simulink model "walnut_1.0"  (R2022a)
settings: Solver=FixedStepAuto  StartTime=0.0  StopTime=inf  RelTol=1e-3
model workspace (MAT data in the model file):
  SL_ROS_VariableLengthArrays_MaxSizes.CommonInfo.ArrayTruncateAction = 'EmitWarning'
  SL_ROS_VariableLengthArrays_MaxSizes.MsgTypeMap = containers.Map
  SL_ROS_VariableLengthArrays_MaxSizes.MsgTypeMap.serialization.keys = {'std_msgs/Float32MultiArray'}
  SL_ROS_VariableLengthArrays_MaxSizes.MsgTypeMap.serialization.values{1}.PropertyName = 'Data'
  SL_ROS_VariableLengthArrays_MaxSizes.MsgTypeMap.serialization.values{1}.DataType = 'single'
  SL_ROS_VariableLengthArrays_MaxSizes.MsgTypeMap.serialization.values{1}.MaxLength = 4
  SL_ROS_VariableLengthArrays_MaxSizes.MsgTypeMap.serialization.uniformity = 0
  SL_ROS_VariableLengthArrays_MaxSizes.MsgTypeMap.serialization.keyType = 'char'
  SL_ROS_VariableLengthArrays_MaxSizes.MsgTypeMap.serialization.valueType = 'any'
  dq0 = [0; 0; 0; 0]
  q0 = [0; 0; 0; 0]
  robotToTest : robotics.RigidBodyTree (value not decoded)
undefined symbols (not defined in the file or in its folder): sawyer, X, Y, Z
libraries: sm_lib x105, nesl_utility x46, robotlib x13, robotmaniplib x6, simulink x5
(part 1 of 3)
settings Model: Creator=conno  LastModifiedBy=conno
settings OptimizationCC: EnhancedBackFolding=on  PassReuseOutputArgsAs=Individual arguments  ZeroExternalMemoryAtStartup=off  ZeroInternalMemoryAtStartup=off  MaxStackSize=64  OptimizeBlockOrder=speed  DifferentSizesBufferReuse=on  OptimizationCustomize=off  EfficientTunableParamExpr=on
settings DebuggingCC: ParameterTunabilityLossMsg=error
settings HardwareCC: ProdBitPerPointer=32  ProdBitPerSizeT=32  ProdBitPerPtrDiffT=32  ProdLargestAtomicFloat=None  ProdIntDivRoundTo=Undefined  ProdEndianess=Unspecified  ProdWordSize=32  ProdHWDeviceType=Generic->Unspecified (assume 32-bit Generic)  UseEmbeddedCoderFeatures=off
settings RTWCC: SystemTargetFile=ert.tlc  HardwareBoard=Robot Operating System (ROS)  TLCOptions="-aInlineSetEventsForThisBaseRateFcn=TLC_FALSE -aSuppressMultiTaskScheduler=TLC_FALSE  -aRateBasedStepFcn=0"  TemplateMakefile=ert_default_tmf  Toolchain=Catkin  TargetLang=C++
settings CodeAppCC: ForceParamTrailComments=on  IgnoreCustomStorageClasses=off  OperatorAnnotations=on  SimulinkDataObjDesc=on  SFDataObjDesc=on  InsertBlockDesc=on
settings ERTTargetCC: SupportNonInlinedSFcns=on

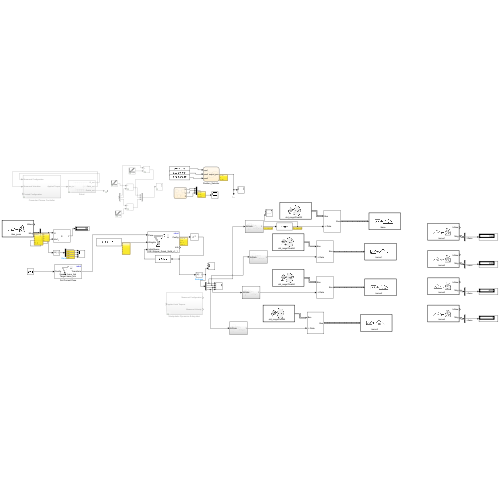
[thumbnail: Simulink's stored preview of the top-level diagram]
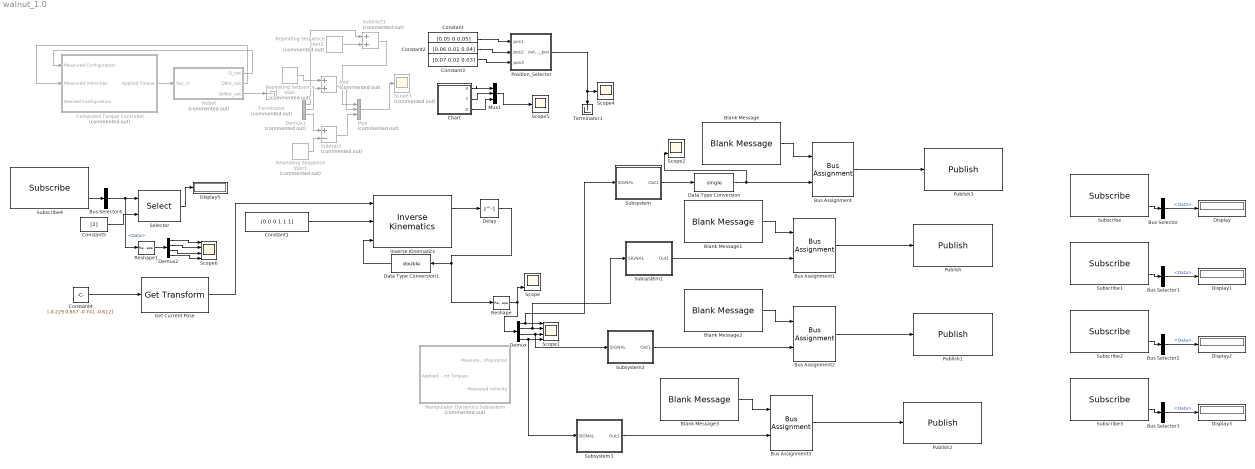
== system walnut_1.0 ==
  Add : Sum  Commented=on
  Blank Message : robotlib/Blank Message  messageClass=Message  entityType=std_msgs/Float32  messageType=std_msgs/Float32  SampleTime=inf  legacyBusStruct=off
  Blank Message1 : robotlib/Blank Message  messageClass=Message  entityType=std_msgs/Float64  messageType=std_msgs/Float64  SampleTime=inf  legacyBusStruct=off
  Blank Message2 : robotlib/Blank Message  messageClass=Message  entityType=std_msgs/Float64  messageType=std_msgs/Float64  SampleTime=inf  legacyBusStruct=off
  Blank Message3 : robotlib/Blank Message  messageClass=Message  entityType=std_msgs/Float64  messageType=std_msgs/Float64  SampleTime=inf  legacyBusStruct=off
  Bus Assignment{,1..3} (4 alike) : BusAssignment  AssignedSignals=Data
  Bus Selector{,1..4} (5 alike) : BusSelector  OutputSignals=Data
  Chart : Stateflow chart  TreatAsAtomicUnit=on
  Computed Torque Controller : Subsystem  Commented=on
  Constant : Constant  Value=[0.05 0 0.05]
  Constant1 : Constant  Value=[0 0 0 1 1 1]
  Constant2 : Constant  Value=[0.06 0.01 0.04]
  Constant3 : Constant  Value=[0.07 0.02 0.03]
  Constant4 : Constant  Value=[-0.229 0.857 -0.741 -0.612]
  Constant5 : Constant  Value=[2]
  Data Type Conversion : DataTypeConversion  OutDataTypeStr=single  SaturateOnIntegerOverflow=off  RndMeth=Floor
  Data Type Conversion1 : DataTypeConversion  OutDataTypeStr=double  SaturateOnIntegerOverflow=off  RndMeth=Floor
  Delay : Delay  DelayLength=1  InitialCondition=q0
  Demux : Demux
  Demux1 : Demux  Commented=on  Outputs=3
  Demux2 : Demux
  Display{,1..3,5} (5 alike) : Display
  Get Current Pose : robotmaniplib/Get Transform  RigidBodyTree=robot  SourceBody=base_link  TargetBody=base_link  SimulateUsing=Interpreted execution
  Inverse Kinematics : robotmaniplib/Inverse Kinematics  RigidBodyTree=robot  EndEffector=Gripper_Dumb_Solid_v1_1  ShowInfo=on  SolverName=BFGS Gradient Projection  EnforceJointLimits=on  MaxIterations=1500  MaxTime=10  GradientTolerance=1e-7  SolutionTolerance=1e-6  StepTolerance=1e-14  ErrorChangeTolerance=1e-12  UseErrorDamping=on  DampingBias=0.0025  SimulateUsing=Interpreted execution
  Manipulator Dynamics Subsystem : Subsystem  Commented=on
  Mux : Mux  Commented=on  Inputs=3
  Mux1 : Mux  Inputs=3
  Position_Selector : Stateflow chart  TreatAsAtomicUnit=on
  Publish : robotlib/Publish  topicSource=Specify your own  topic=/servo1  messageType=std_msgs/Float64  legacyBusStruct=off  messageQueueLength=1
  Publish1 : robotlib/Publish  topicSource=Specify your own  topic=/servo2  messageType=std_msgs/Float64  legacyBusStruct=off  messageQueueLength=1
  Publish2 : robotlib/Publish  topicSource=Specify your own  topic=/servo3  messageType=std_msgs/Float64  legacyBusStruct=off  messageQueueLength=1
  Publish3 : robotlib/Publish  topicSource=Specify your own  topic=/base  messageType=std_msgs/Float32  legacyBusStruct=off  messageQueueLength=1
  Repeating Sequence Stair : simulink/Sources/Repeating Sequence Stair  Commented=on  OutValues=[0 0.01 0.02 0.03].'  tsamp=2  OutMin=[]  OutMax=[]  OutDataTypeStr=double  OutputDataTypeScalingMode=double  OutDataType=fixdt(0,8)  ConRadixGroup=Best Precision: Vector-wise  OutScaling=2^-12
  Repeating Sequence Stair1 : simulink/Sources/Repeating Sequence Stair  Commented=on  OutValues=[0 0.01 0.02 0.03].'  tsamp=2  OutMin=[]  OutMax=[]  OutDataTypeStr=double  OutputDataTypeScalingMode=double  OutDataType=fixdt(0,8)  ConRadixGroup=Best Precision: Vector-wise  OutScaling=2^-12
  Repeating Sequence Stair2 : simulink/Sources/Repeating Sequence Stair  Commented=on  OutValues=[0 0.01 0.02 0.03].'  tsamp=2  OutMin=[]  OutMax=[]  OutDataTypeStr=double  OutputDataTypeScalingMode=double  OutDataType=fixdt(0,8)  ConRadixGroup=Best Precision: Vector-wise  OutScaling=2^-12
  Reshape : Reshape
  Reshape1 : Reshape
  Robot : Subsystem  Commented=on
  Scope : Scope  NumInputPorts=3
  Scope1 : Scope  NumInputPorts=4
  Scope2 : Scope  NumInputPorts=3
  Scope3 : Scope  Commented=on
  Scope4 : Scope
  Scope5 : Scope
  Scope6 : Scope  NumInputPorts=4
  Selector : Selector  IndexOptions=Index vector (port)  Indices=[2]  OutputSizes=1
  Subscribe : robotlib/Subscribe  topicSource=Specify your own  topic=/servo1  messageType=std_msgs/Float64  SampleTime=-1  legacyBusStruct=off  messageQueueLength=1
  Subscribe1 : robotlib/Subscribe  topicSource=Specify your own  topic=/servo2  messageType=std_msgs/Float64  SampleTime=-1  legacyBusStruct=off  messageQueueLength=1
  Subscribe2 : robotlib/Subscribe  topicSource=Specify your own  topic=/servo3  messageType=std_msgs/Float64  SampleTime=-1  legacyBusStruct=off  messageQueueLength=1
  Subscribe3 : robotlib/Subscribe  topicSource=Specify your own  topic=/servo4  messageType=std_msgs/Float64  SampleTime=-1  legacyBusStruct=off  messageQueueLength=1
  Subscribe4 : robotlib/Subscribe  topicSource=Select from ROS network  topic=/des_pose  messageType=std_msgs/Float32MultiArray  SampleTime=-1  legacyBusStruct=off  messageQueueLength=1
  Subsystem : Subsystem
  Subsystem1 : Subsystem
  Subsystem2 : Subsystem
  Subsystem3 : Subsystem
  Subtract : Sum  Commented=on  Inputs=+-
  Subtract1 : Sum  Commented=on
  Terminator : Terminator  Commented=on
  Terminator1 : Terminator
  wires:
  Bus Selector3/1 -> Display3/1  "<Data>"
  Subscribe3/2 -> Bus Selector3/1
  Subscribe1/2 -> Bus Selector1/1
  Reshape/1 -> Scope/3, Demux/1
  Computed Torque Controller/1(Applied Torque) -> Robot/1(tau_in)
  Demux/1 -> Subsystem/1(SIGNAL), Scope1/1
  Bus Assignment2/1 -> Publish1/1
  Blank Message1/1 -> Bus Assignment1/1
  Blank Message2/1 -> Bus Assignment2/1
  Bus Assignment1/1 -> Publish/1
  Bus Assignment3/1 -> Publish2/1
  Subscribe2/2 -> Bus Selector2/1
  Bus Selector2/1 -> Display2/1  "<Data>"
  Get Current Pose/1 -> Inverse Kinematics/1
  Inverse Kinematics/1 -> Delay/1
  Bus Selector/1 -> Display/1  "<Data>"
  Subscribe/2 -> Bus Selector/1
  Blank Message3/1 -> Bus Assignment3/1
  Demux/4 -> Subsystem3/1(SIGNAL), Scope1/4
  Robot/1(Q_out) -> Computed Torque Controller/1(Measured Configuration)
  Bus Selector1/1 -> Display1/1  "<Data>"
  Constant1/1 -> Inverse Kinematics/2
  Demux/3 -> Subsystem2/1(SIGNAL), Scope1/3
  Bus Assignment/1 -> Publish3/1
  Demux/2 -> Subsystem1/1(SIGNAL), Scope1/2
  Robot/2(Qdot_out) -> Computed Torque Controller/2(Measured Velocities)
  Robot/3(Qddot_out) -> Terminator/1
  Blank Message/1 -> Bus Assignment/1
  Delay/1 -> Reshape/1, Data Type Conversion1/1
  Subsystem/1(Out1) -> Data Type Conversion/1
  Subsystem1/1(Out1) -> Bus Assignment1/2
  Subsystem2/1(Out1) -> Bus Assignment2/2
  Subsystem3/1(Out1) -> Bus Assignment3/2
  Repeating Sequence Stair/1 -> Add/1
  Add/1 -> Mux/2
  Mux/1 -> Scope3/1
  Demux1/1 -> Subtract1/1
  Demux1/2 -> Add/2
  Demux1/3 -> Subtract/1
  Repeating Sequence Stair1/1 -> Subtract/2
  Subtract/1 -> Mux/3
  Repeating Sequence Stair2/1 -> Subtract1/2
  Subtract1/1 -> Mux/1
  Constant/1 -> Position_Selector/1(pos1)
  Constant2/1 -> Position_Selector/2(pos2)
  Constant3/1 -> Position_Selector/3(pos3)
  Position_Selector/1(output_pos) -> Terminator1/1, Scope4/1
  Chart/1(X) -> Mux1/1
  Chart/2(Y) -> Mux1/2
  Chart/3(Z) -> Mux1/3
  Mux1/1 -> Scope5/1
  Data Type Conversion/1 -> Scope2/3, Bus Assignment/2
  Data Type Conversion1/1 -> Inverse Kinematics/3
  Constant4/1 -> Get Current Pose/1
  Subscribe4/2 -> Bus Selector4/1
  Bus Selector4/1 -> Reshape1/1, Selector/1  "<Data>"
  Constant5/1 -> Selector/2
  Selector/1 -> Display5/1
  Demux2/1 -> Scope6/1
  Demux2/2 -> Scope6/2
  Demux2/3 -> Scope6/3
  Demux2/4 -> Scope6/4
  Reshape1/1 -> Demux2/1

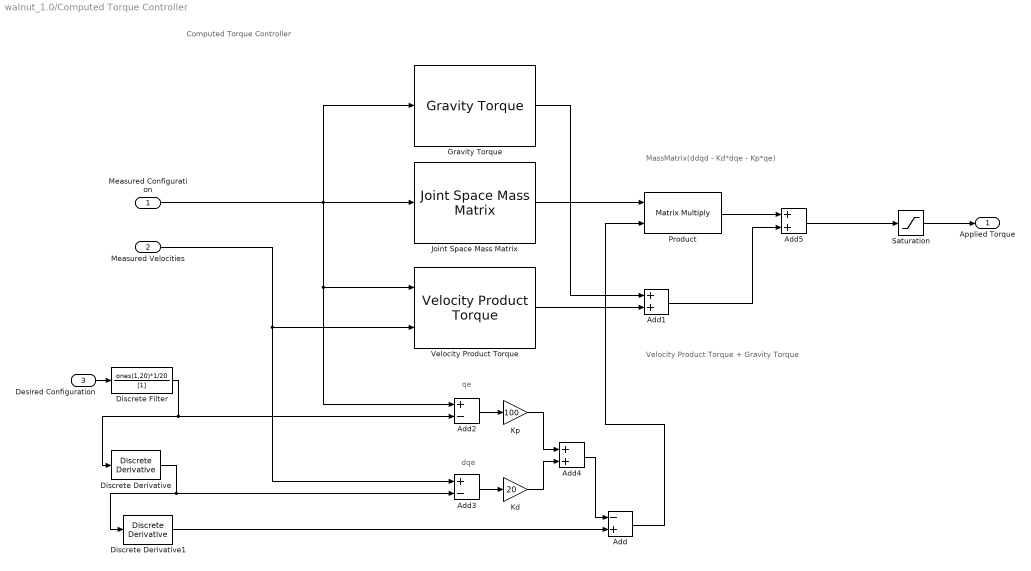
== system walnut_1.0/Computed Torque Controller ==
  note: Computed Torque Controller
  note: MassMatrix(ddqd - Kd*dqe - Kp*qe)
  note: Velocity Product Torque + Gravity Torque
  note: dqe
  note: qe
  Measured Configuration : Inport
  Measured Velocities : Inport  Port=2
  Desired Configuration : Inport  Port=3
  Add : Sum  Inputs=-+
  Add1 : Sum
  Add2 : Sum  Inputs=+-
  Add3 : Sum  Inputs=+-
  Add4 : Sum
  Add5 : Sum
  Discrete Derivative : simulink/Discrete/Discrete Derivative  gainval=1.0  ICPrevScaledInput=0.0  OutMin=[]  OutMax=[]  OutDataType=fixdt(1, 16)  OutScaling=2^-10  DoSatur=off
  Discrete Derivative1 : simulink/Discrete/Discrete Derivative  gainval=1.0  ICPrevScaledInput=0.0  OutMin=[]  OutMax=[]  OutDataType=fixdt(1, 16)  OutScaling=2^-10  DoSatur=off
  Discrete Filter : DiscreteFilter  Numerator=ones(1,20)*1/20  Denominator=[1]  InitialStates=repmat(q0',19,1)
  Gravity Torque : robotmaniplib/Gravity Torque  RigidBodyTree=robot  SimulateUsing=Interpreted execution
  Joint Space Mass Matrix : robotmaniplib/Joint Space Mass Matrix  RigidBodyTree=robot  SimulateUsing=Interpreted execution
  Kd : Gain  Gain=20
  Kp : Gain  Gain=100
  Product : Product  Multiplication=Matrix(*)
  Saturation : Saturate  UpperLimit=100  LowerLimit=-100
  Velocity Product Torque : robotmaniplib/Velocity Product Torque  RigidBodyTree=robot  SimulateUsing=Interpreted execution
      settings: SourceProductBaseCode=RO
  Applied Torque : Outport  VectorParamsAs1DForOutWhenUnconnected=off
  wires:
  Saturation/1 -> Applied Torque/1
  Velocity Product Torque/1 -> Add1/2
  Gravity Torque/1 -> Add1/1
  Add1/1 -> Add5/2
  Product/1 -> Add5/1
  Add5/1 -> Saturation/1
  Kd/1 -> Add4/2
  Kp/1 -> Add4/1
  Add3/1 -> Kd/1
  Add2/1 -> Kp/1
  Discrete Derivative/1 -> Discrete Derivative1/1, Add3/2
  Desired Configuration/1 -> Discrete Filter/1
  Add/1 -> Product/2
  Discrete Derivative1/1 -> Add/2
  Add4/1 -> Add/1
  Measured Velocities/1 -> Velocity Product Torque/2, Add3/1
  Measured Configuration/1 -> Add2/1, Velocity Product Torque/1, Gravity Torque/1, Joint Space Mass Matrix/1
  Joint Space Mass Matrix/1 -> Product/1
  Discrete Filter/1 -> Discrete Derivative/1, Add2/2

== system walnut_1.0/Manipulator Dynamics Subsystem ==
  Applied Joint Torques : Inport
  Integrator : Integrator
  Integrator1 : Integrator  InitialCondition=q0
  Manipulator Dynamics Model : robotmaniplib/Forward Dynamics  RigidBodyTree=robot  SimulateUsing=Interpreted execution
  Zero : Constant  Value=zeros(6, sawyer.NumBodies)  OutDataTypeStr=Inherit: Inherit via back propagation
  Measured Configuration : Outport  VectorParamsAs1DForOutWhenUnconnected=off
  Measured Velocity : Outport  Port=2  VectorParamsAs1DForOutWhenUnconnected=off
  wires:
  Integrator1/1 -> Manipulator Dynamics Model/1, Measured Configuration/1
  Manipulator Dynamics Model/1 -> Integrator/1
  Integrator/1 -> Integrator1/1, Manipulator Dynamics Model/2, Measured Velocity/1
  Applied Joint Torques/1 -> Manipulator Dynamics Model/3
  Zero/1 -> Manipulator Dynamics Model/4

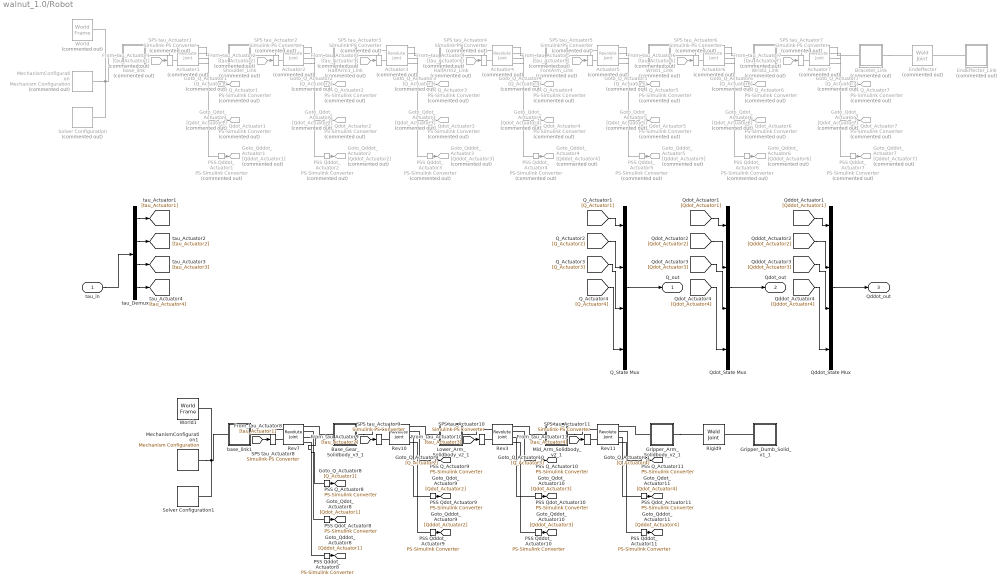
== system walnut_1.0/Robot ==
  tau_in : Inport
  Actuator1 : sm_lib/Joints/Revolute Joint  Commented=on  JointMode=Normal  SenseConstraintForce=off  SenseConstraintForceX=off  SenseConstraintForceY=off  SenseConstraintForceZ=off  SenseConstraintTorque=off  SenseConstraintTorqueX=off  SenseConstraintTorqueY=off  SenseConstraintTorqueZ=off  SenseTotalForce=off  SenseTotalForceX=off  SenseTotalForceY=off  SenseTotalForceZ=off  SenseTotalTorque=off  SenseTotalTorqueX=off  SenseTotalTorqueY=off  SenseTotalTorqueZ=off  CompositeWrenchDir=FollowerOnBase  CompositeWrenchFrame=BaseFrame  EquilibriumPosition=0  EquilibriumPositionUnits=deg  SpringStiffness=0  SpringStiffnessUnits=N*m/deg  DampingCoefficient=0  DampingCoefficientUnits=kg*m^2/(rad*s)  TorqueActuationMode=InputTorque  MotionActuationMode=ComputedMotion  SensePosition=on  SenseVelocity=on  SenseAcceleration=on  SenseTorqueForce=off  SenseLowerLimitTorqueForce=off  SenseUpperLimitTorqueForce=off  LowerLimitSpecify=off  LowerLimitBound=-90  LowerLimitBoundUnits=deg  LowerLimitStiffness=1e4  LowerLimitStiffnessUnits=N*m/deg  LowerLimitDamping=10  LowerLimitDampingUnits=N*m/(deg/s)  LowerLimitTransitionRegionWidth=0.1  LowerLimitTransitionRegionWidthUnits=deg  UpperLimitSpecify=off  UpperLimitBound=90  UpperLimitBoundUnits=deg  UpperLimitStiffness=1e4  UpperLimitStiffnessUnits=N*m/deg  UpperLimitDamping=10  UpperLimitDampingUnits=N*m/(deg/s)  UpperLimitTransitionRegionWidth=0.1  UpperLimitTransitionRegionWidthUnits=deg  PositionTargetSpecify=on  PositionTargetPriority=High  PositionTargetValue=q0(1)  PositionTargetValueUnits=rad  VelocityTargetSpecify=on  VelocityTargetPriority=High  VelocityTargetValue=dq0(1)  VelocityTargetValueUnits=rad/s
  Actuator2 : sm_lib/Joints/Revolute Joint  Commented=on  JointMode=Normal  SenseConstraintForce=off  SenseConstraintForceX=off  SenseConstraintForceY=off  SenseConstraintForceZ=off  SenseConstraintTorque=off  SenseConstraintTorqueX=off  SenseConstraintTorqueY=off  SenseConstraintTorqueZ=off  SenseTotalForce=off  SenseTotalForceX=off  SenseTotalForceY=off  SenseTotalForceZ=off  SenseTotalTorque=off  SenseTotalTorqueX=off  SenseTotalTorqueY=off  SenseTotalTorqueZ=off  CompositeWrenchDir=FollowerOnBase  CompositeWrenchFrame=BaseFrame  EquilibriumPosition=0  EquilibriumPositionUnits=deg  SpringStiffness=0  SpringStiffnessUnits=N*m/deg  DampingCoefficient=0  DampingCoefficientUnits=kg*m^2/(rad*s)  TorqueActuationMode=InputTorque  MotionActuationMode=ComputedMotion  SensePosition=on  SenseVelocity=on  SenseAcceleration=on  SenseTorqueForce=off  SenseLowerLimitTorqueForce=off  SenseUpperLimitTorqueForce=off  LowerLimitSpecify=on  LowerLimitBound=-2.2  LowerLimitBoundUnits=rad  LowerLimitStiffness=1e4  LowerLimitStiffnessUnits=N*m/deg  LowerLimitDamping=10  LowerLimitDampingUnits=N*m/(deg/s)  LowerLimitTransitionRegionWidth=0.1  LowerLimitTransitionRegionWidthUnits=deg  UpperLimitSpecify=on  UpperLimitBound=2.2  UpperLimitBoundUnits=rad  UpperLimitStiffness=1e4  UpperLimitStiffnessUnits=N*m/deg  UpperLimitDamping=10  UpperLimitDampingUnits=N*m/(deg/s)  UpperLimitTransitionRegionWidth=0.1  UpperLimitTransitionRegionWidthUnits=deg  PositionTargetSpecify=on  PositionTargetPriority=High  PositionTargetValue=q0(2)  PositionTargetValueUnits=rad  VelocityTargetSpecify=on  VelocityTargetPriority=High  VelocityTargetValue=dq0(2)  VelocityTargetValueUnits=rad/s
  Actuator3 : sm_lib/Joints/Revolute Joint  Commented=on  JointMode=Normal  SenseConstraintForce=off  SenseConstraintForceX=off  SenseConstraintForceY=off  SenseConstraintForceZ=off  SenseConstraintTorque=off  SenseConstraintTorqueX=off  SenseConstraintTorqueY=off  SenseConstraintTorqueZ=off  SenseTotalForce=off  SenseTotalForceX=off  SenseTotalForceY=off  SenseTotalForceZ=off  SenseTotalTorque=off  SenseTotalTorqueX=off  SenseTotalTorqueY=off  SenseTotalTorqueZ=off  CompositeWrenchDir=FollowerOnBase  CompositeWrenchFrame=BaseFrame  EquilibriumPosition=0  EquilibriumPositionUnits=deg  SpringStiffness=0  SpringStiffnessUnits=N*m/deg  DampingCoefficient=0  DampingCoefficientUnits=kg*m^2/(rad*s)  TorqueActuationMode=InputTorque  MotionActuationMode=ComputedMotion  SensePosition=on  SenseVelocity=on  SenseAcceleration=on  SenseTorqueForce=off  SenseLowerLimitTorqueForce=off  SenseUpperLimitTorqueForce=off  LowerLimitSpecify=off  LowerLimitBound=-90  LowerLimitBoundUnits=deg  LowerLimitStiffness=1e4  LowerLimitStiffnessUnits=N*m/deg  LowerLimitDamping=10  LowerLimitDampingUnits=N*m/(deg/s)  LowerLimitTransitionRegionWidth=0.1  LowerLimitTransitionRegionWidthUnits=deg  UpperLimitSpecify=off  UpperLimitBound=90  UpperLimitBoundUnits=deg  UpperLimitStiffness=1e4  UpperLimitStiffnessUnits=N*m/deg  UpperLimitDamping=10  UpperLimitDampingUnits=N*m/(deg/s)  UpperLimitTransitionRegionWidth=0.1  UpperLimitTransitionRegionWidthUnits=deg  PositionTargetSpecify=on  PositionTargetPriority=High  PositionTargetValue=q0(3)  PositionTargetValueUnits=rad  VelocityTargetSpecify=on  VelocityTargetPriority=High  VelocityTargetValue=dq0(3)  VelocityTargetValueUnits=rad/s
  Actuator4 : sm_lib/Joints/Revolute Joint  Commented=on  JointMode=Normal  SenseConstraintForce=off  SenseConstraintForceX=off  SenseConstraintForceY=off  SenseConstraintForceZ=off  SenseConstraintTorque=off  SenseConstraintTorqueX=off  SenseConstraintTorqueY=off  SenseConstraintTorqueZ=off  SenseTotalForce=off  SenseTotalForceX=off  SenseTotalForceY=off  SenseTotalForceZ=off  SenseTotalTorque=off  SenseTotalTorqueX=off  SenseTotalTorqueY=off  SenseTotalTorqueZ=off  CompositeWrenchDir=FollowerOnBase  CompositeWrenchFrame=BaseFrame  EquilibriumPosition=0  EquilibriumPositionUnits=deg  SpringStiffness=0  SpringStiffnessUnits=N*m/deg  DampingCoefficient=0  DampingCoefficientUnits=kg*m^2/(rad*s)  TorqueActuationMode=InputTorque  MotionActuationMode=ComputedMotion  SensePosition=on  SenseVelocity=on  SenseAcceleration=on  SenseTorqueForce=off  SenseLowerLimitTorqueForce=off  SenseUpperLimitTorqueForce=off  LowerLimitSpecify=on  LowerLimitBound=-2.5656  LowerLimitBoundUnits=rad  LowerLimitStiffness=1e4  LowerLimitStiffnessUnits=N*m/deg  LowerLimitDamping=10  LowerLimitDampingUnits=N*m/(deg/s)  LowerLimitTransitionRegionWidth=0.1  LowerLimitTransitionRegionWidthUnits=deg  UpperLimitSpecify=on  UpperLimitBound=2.5656  UpperLimitBoundUnits=rad  UpperLimitStiffness=1e4  UpperLimitStiffnessUnits=N*m/deg  UpperLimitDamping=10  UpperLimitDampingUnits=N*m/(deg/s)  UpperLimitTransitionRegionWidth=0.1  UpperLimitTransitionRegionWidthUnits=deg  PositionTargetSpecify=on  PositionTargetPriority=High  PositionTargetValue=q0(4)  PositionTargetValueUnits=rad  VelocityTargetSpecify=on  VelocityTargetPriority=High  VelocityTargetValue=dq0(4)  VelocityTargetValueUnits=rad/s
  Actuator5 : sm_lib/Joints/Revolute Joint  Commented=on  JointMode=Normal  SenseConstraintForce=off  SenseConstraintForceX=off  SenseConstraintForceY=off  SenseConstraintForceZ=off  SenseConstraintTorque=off  SenseConstraintTorqueX=off  SenseConstraintTorqueY=off  SenseConstraintTorqueZ=off  SenseTotalForce=off  SenseTotalForceX=off  SenseTotalForceY=off  SenseTotalForceZ=off  SenseTotalTorque=off  SenseTotalTorqueX=off  SenseTotalTorqueY=off  SenseTotalTorqueZ=off  CompositeWrenchDir=FollowerOnBase  CompositeWrenchFrame=BaseFrame  EquilibriumPosition=0  EquilibriumPositionUnits=deg  SpringStiffness=0  SpringStiffnessUnits=N*m/deg  DampingCoefficient=0  DampingCoefficientUnits=kg*m^2/(rad*s)  TorqueActuationMode=InputTorque  MotionActuationMode=ComputedMotion  SensePosition=on  SenseVelocity=on  SenseAcceleration=on  SenseTorqueForce=off  SenseLowerLimitTorqueForce=off  SenseUpperLimitTorqueForce=off  LowerLimitSpecify=off  LowerLimitBound=-90  LowerLimitBoundUnits=deg  LowerLimitStiffness=1e4  LowerLimitStiffnessUnits=N*m/deg  LowerLimitDamping=10  LowerLimitDampingUnits=N*m/(deg/s)  LowerLimitTransitionRegionWidth=0.1  LowerLimitTransitionRegionWidthUnits=deg  UpperLimitSpecify=off  UpperLimitBound=90  UpperLimitBoundUnits=deg  UpperLimitStiffness=1e4  UpperLimitStiffnessUnits=N*m/deg  UpperLimitDamping=10  UpperLimitDampingUnits=N*m/(deg/s)  UpperLimitTransitionRegionWidth=0.1  UpperLimitTransitionRegionWidthUnits=deg  PositionTargetSpecify=on  PositionTargetPriority=High  PositionTargetValue=q0(5)  PositionTargetValueUnits=rad  VelocityTargetSpecify=on  VelocityTargetPriority=High  VelocityTargetValue=dq0(5)  VelocityTargetValueUnits=rad/s
  Actuator6 : sm_lib/Joints/Revolute Joint  Commented=on  JointMode=Normal  SenseConstraintForce=off  SenseConstraintForceX=off  SenseConstraintForceY=off  SenseConstraintForceZ=off  SenseConstraintTorque=off  SenseConstraintTorqueX=off  SenseConstraintTorqueY=off  SenseConstraintTorqueZ=off  SenseTotalForce=off  SenseTotalForceX=off  SenseTotalForceY=off  SenseTotalForceZ=off  SenseTotalTorque=off  SenseTotalTorqueX=off  SenseTotalTorqueY=off  SenseTotalTorqueZ=off  CompositeWrenchDir=FollowerOnBase  CompositeWrenchFrame=BaseFrame  EquilibriumPosition=0  EquilibriumPositionUnits=deg  SpringStiffness=0  SpringStiffnessUnits=N*m/deg  DampingCoefficient=0  DampingCoefficientUnits=kg*m^2/(rad*s)  TorqueActuationMode=InputTorque  MotionActuationMode=ComputedMotion  SensePosition=on  SenseVelocity=on  SenseAcceleration=on  SenseTorqueForce=off  SenseLowerLimitTorqueForce=off  SenseUpperLimitTorqueForce=off  LowerLimitSpecify=on  LowerLimitBound=-2.05  LowerLimitBoundUnits=rad  LowerLimitStiffness=1e4  LowerLimitStiffnessUnits=N*m/deg  LowerLimitDamping=10  LowerLimitDampingUnits=N*m/(deg/s)  LowerLimitTransitionRegionWidth=0.1  LowerLimitTransitionRegionWidthUnits=deg  UpperLimitSpecify=on  UpperLimitBound=2.05  UpperLimitBoundUnits=rad  UpperLimitStiffness=1e4  UpperLimitStiffnessUnits=N*m/deg  UpperLimitDamping=10  UpperLimitDampingUnits=N*m/(deg/s)  UpperLimitTransitionRegionWidth=0.1  UpperLimitTransitionRegionWidthUnits=deg  PositionTargetSpecify=on  PositionTargetPriority=High  PositionTargetValue=q0(6)  PositionTargetValueUnits=rad  VelocityTargetSpecify=on  VelocityTargetPriority=High  VelocityTargetValue=dq0(6)  VelocityTargetValueUnits=rad/s
  Actuator7 : sm_lib/Joints/Revolute Joint  Commented=on  JointMode=Normal  SenseConstraintForce=off  SenseConstraintForceX=off  SenseConstraintForceY=off  SenseConstraintForceZ=off  SenseConstraintTorque=off  SenseConstraintTorqueX=off  SenseConstraintTorqueY=off  SenseConstraintTorqueZ=off  SenseTotalForce=off  SenseTotalForceX=off  SenseTotalForceY=off  SenseTotalForceZ=off  SenseTotalTorque=off  SenseTotalTorqueX=off  SenseTotalTorqueY=off  SenseTotalTorqueZ=off  CompositeWrenchDir=FollowerOnBase  CompositeWrenchFrame=BaseFrame  EquilibriumPosition=0  EquilibriumPositionUnits=deg  SpringStiffness=0  SpringStiffnessUnits=N*m/deg  DampingCoefficient=0  DampingCoefficientUnits=kg*m^2/(rad*s)  TorqueActuationMode=InputTorque  MotionActuationMode=ComputedMotion  SensePosition=on  SenseVelocity=on  SenseAcceleration=on  SenseTorqueForce=off  SenseLowerLimitTorqueForce=off  SenseUpperLimitTorqueForce=off  LowerLimitSpecify=off  LowerLimitBound=-90  LowerLimitBoundUnits=deg  LowerLimitStiffness=1e4  LowerLimitStiffnessUnits=N*m/deg  LowerLimitDamping=10  LowerLimitDampingUnits=N*m/(deg/s)  LowerLimitTransitionRegionWidth=0.1  LowerLimitTransitionRegionWidthUnits=deg  UpperLimitSpecify=off  UpperLimitBound=90  UpperLimitBoundUnits=deg  UpperLimitStiffness=1e4  UpperLimitStiffnessUnits=N*m/deg  UpperLimitDamping=10  UpperLimitDampingUnits=N*m/(deg/s)  UpperLimitTransitionRegionWidth=0.1  UpperLimitTransitionRegionWidthUnits=deg  PositionTargetSpecify=on  PositionTargetPriority=High  PositionTargetValue=q0(7)  PositionTargetValueUnits=rad  VelocityTargetSpecify=on  VelocityTargetPriority=High  VelocityTargetValue=dq0(7)  VelocityTargetValueUnits=rad/s
  Base_Gear_Solidbody_v3_1 : Subsystem
  Bracelet_Link : Subsystem  Commented=on
  EndEffector_Link : Subsystem  Commented=on
  Endeffector : sm_lib/Joints/Weld Joint  Commented=on  JointMode=Normal  SenseConstraintForce=off  SenseConstraintForceX=off  SenseConstraintForceY=off  SenseConstraintForceZ=off  SenseConstraintTorque=off  SenseConstraintTorqueX=off  SenseConstraintTorqueY=off  SenseConstraintTorqueZ=off  SenseTotalForce=off  SenseTotalForceX=off  SenseTotalForceY=off  SenseTotalForceZ=off  SenseTotalTorque=off  SenseTotalTorqueX=off  SenseTotalTorqueY=off  SenseTotalTorqueZ=off  CompositeWrenchDir=FollowerOnBase  CompositeWrenchFrame=BaseFrame
  ForeArm_Link : Subsystem  Commented=on
  From_tau_Actuator1 : From  Commented=on  GotoTag=tau_Actuator1
  From_tau_Actuator2 : From  Commented=on  GotoTag=tau_Actuator2
  From_tau_Actuator3 : From  Commented=on  GotoTag=tau_Actuator3
  From_tau_Actuator4 : From  Commented=on  GotoTag=tau_Actuator4
  From_tau_Actuator5 : From  Commented=on  GotoTag=tau_Actuator5
  From_tau_Actuator6 : From  Commented=on  GotoTag=tau_Actuator6
  From_tau_Actuator7 : From  Commented=on  GotoTag=tau_Actuator7
  Goto_Q_Actuator1 : Goto  Commented=on  GotoTag=Q_Actuator1
  Goto_Q_Actuator2 : Goto  Commented=on  GotoTag=Q_Actuator2
  Goto_Q_Actuator3 : Goto  Commented=on  GotoTag=Q_Actuator3
  Goto_Q_Actuator4 : Goto  Commented=on  GotoTag=Q_Actuator4
  Goto_Q_Actuator5 : Goto  Commented=on  GotoTag=Q_Actuator5
  Goto_Q_Actuator6 : Goto  Commented=on  GotoTag=Q_Actuator6
  Goto_Q_Actuator7 : Goto  Commented=on  GotoTag=Q_Actuator7
  Goto_Qddot_Actuator1 : Goto  Commented=on  GotoTag=Qddot_Actuator1
  Goto_Qddot_Actuator2 : Goto  Commented=on  GotoTag=Qddot_Actuator2
  Goto_Qddot_Actuator3 : Goto  Commented=on  GotoTag=Qddot_Actuator3
  Goto_Qddot_Actuator4 : Goto  Commented=on  GotoTag=Qddot_Actuator4
  Goto_Qddot_Actuator5 : Goto  Commented=on  GotoTag=Qddot_Actuator5
  Goto_Qddot_Actuator6 : Goto  Commented=on  GotoTag=Qddot_Actuator6
  Goto_Qddot_Actuator7 : Goto  Commented=on  GotoTag=Qddot_Actuator7
  Goto_Qdot_Actuator1 : Goto  Commented=on  GotoTag=Qdot_Actuator1
  Goto_Qdot_Actuator2 : Goto  Commented=on  GotoTag=Qdot_Actuator2
  Goto_Qdot_Actuator3 : Goto  Commented=on  GotoTag=Qdot_Actuator3
  Goto_Qdot_Actuator4 : Goto  Commented=on  GotoTag=Qdot_Actuator4
  Goto_Qdot_Actuator5 : Goto  Commented=on  GotoTag=Qdot_Actuator5
  Goto_Qdot_Actuator6 : Goto  Commented=on  GotoTag=Qdot_Actuator6
  Goto_Qdot_Actuator7 : Goto  Commented=on  GotoTag=Qdot_Actuator7
  Gripper_Arm_Solidbody_v2_1 : Subsystem
  Gripper_Dumb_Solid_v1_1 : Subsystem
  HalfArm1_Link : Subsystem  Commented=on
  HalfArm2_Link : Subsystem  Commented=on
  Lower_Arm_Solidbody_v2_1 : Subsystem
  MechanismConfiguration : sm_lib/Utilities/Mechanism Configuration  Commented=on  UniformGravity=Constant  GravityVector=[0, 0, 0]  GravityUnits=m/s^2  LinearizationDelta=0.001  JointModeTransitionNonlinearIterations=2
  MechanismConfiguration1 : sm_lib/Utilities/Mechanism Configuration  UniformGravity=Constant  GravityVector=[0, 0, 0]  GravityUnits=m/s^2  LinearizationDelta=0.001  JointModeTransitionNonlinearIterations=2
  Mid_Arm_Solidbody_v2_1 : Subsystem
  PSS Q_Actuator{1..7} (7 alike) : nesl_utility/PS-Simulink Converter  Commented=on  PhysicalDomain=network_engine_domain  SubClassName=ps_output  LeftPortType=input  RightPortType=output  PseudoPeriodic=off  Frequencies=[]  VectorFormat=inherit  Unit=inherit  AffineConversion=off
      settings: SourceProductBaseCode=SS,PW,VE
  PSS Q_Actuator{8..11} (4 alike) : nesl_utility/PS-Simulink Converter  PhysicalDomain=network_engine_domain  SubClassName=ps_output  LeftPortType=input  RightPortType=output  PseudoPeriodic=off  Frequencies=[]  VectorFormat=inherit  Unit=inherit  AffineConversion=off
      settings: SourceProductBaseCode=SS,PW,VE
  PSS Qddot_Actuator{1..7} (7 alike) : nesl_utility/PS-Simulink Converter  Commented=on  PhysicalDomain=network_engine_domain  SubClassName=ps_output  LeftPortType=input  RightPortType=output  PseudoPeriodic=off  Frequencies=[]  VectorFormat=inherit  Unit=inherit  AffineConversion=off
      settings: SourceProductBaseCode=SS,PW,VE
  PSS Qddot_Actuator{8..11} (4 alike) : nesl_utility/PS-Simulink Converter  PhysicalDomain=network_engine_domain  SubClassName=ps_output  LeftPortType=input  RightPortType=output  PseudoPeriodic=off  Frequencies=[]  VectorFormat=inherit  Unit=inherit  AffineConversion=off
      settings: SourceProductBaseCode=SS,PW,VE
  PSS Qdot_Actuator{1..7} (7 alike) : nesl_utility/PS-Simulink Converter  Commented=on  PhysicalDomain=network_engine_domain  SubClassName=ps_output  LeftPortType=input  RightPortType=output  PseudoPeriodic=off  Frequencies=[]  VectorFormat=inherit  Unit=inherit  AffineConversion=off
      settings: SourceProductBaseCode=SS,PW,VE
  PSS Qdot_Actuator{8..11} (4 alike) : nesl_utility/PS-Simulink Converter  PhysicalDomain=network_engine_domain  SubClassName=ps_output  LeftPortType=input  RightPortType=output  PseudoPeriodic=off  Frequencies=[]  VectorFormat=inherit  Unit=inherit  AffineConversion=off
      settings: SourceProductBaseCode=SS,PW,VE
  Q_State Mux : Mux
  Qddot_State Mux : Mux
  Qdot_State Mux : Mux
  Rev10 : sm_lib/Joints/Revolute Joint  JointMode=Normal  SenseConstraintForce=off  SenseConstraintForceX=off  SenseConstraintForceY=off  SenseConstraintForceZ=off  SenseConstraintTorque=off  SenseConstraintTorqueX=off  SenseConstraintTorqueY=off  SenseConstraintTorqueZ=off  SenseTotalForce=off  SenseTotalForceX=off  SenseTotalForceY=off  SenseTotalForceZ=off  SenseTotalTorque=off  SenseTotalTorqueX=off  SenseTotalTorqueY=off  SenseTotalTorqueZ=off  CompositeWrenchDir=FollowerOnBase  CompositeWrenchFrame=BaseFrame  EquilibriumPosition=0  EquilibriumPositionUnits=deg  SpringStiffness=0  SpringStiffnessUnits=N*m/deg  DampingCoefficient=0  DampingCoefficientUnits=kg*m^2/(rad*s)  TorqueActuationMode=InputTorque  MotionActuationMode=ComputedMotion  SensePosition=on  SenseVelocity=on  SenseAcceleration=on  SenseTorqueForce=off  SenseLowerLimitTorqueForce=off  SenseUpperLimitTorqueForce=off  LowerLimitSpecify=on  LowerLimitBound=-1.57  LowerLimitBoundUnits=rad  LowerLimitStiffness=1e4  LowerLimitStiffnessUnits=N*m/deg  LowerLimitDamping=10  LowerLimitDampingUnits=N*m/(deg/s)  LowerLimitTransitionRegionWidth=0.1  LowerLimitTransitionRegionWidthUnits=deg  UpperLimitSpecify=on  UpperLimitBound=1.2  UpperLimitBoundUnits=rad  UpperLimitStiffness=1e4  UpperLimitStiffnessUnits=N*m/deg  UpperLimitDamping=10  UpperLimitDampingUnits=N*m/(deg/s)  UpperLimitTransitionRegionWidth=0.1  UpperLimitTransitionRegionWidthUnits=deg  PositionTargetSpecify=on  PositionTargetPriority=High  PositionTargetValue=q0(2)  PositionTargetValueUnits=rad  VelocityTargetSpecify=on  VelocityTargetPriority=High  VelocityTargetValue=dq0(2)  VelocityTargetValueUnits=rad/s
  Rev11 : sm_lib/Joints/Revolute Joint  JointMode=Normal  SenseConstraintForce=off  SenseConstraintForceX=off  SenseConstraintForceY=off  SenseConstraintForceZ=off  SenseConstraintTorque=off  SenseConstraintTorqueX=off  SenseConstraintTorqueY=off  SenseConstraintTorqueZ=off  SenseTotalForce=off  SenseTotalForceX=off  SenseTotalForceY=off  SenseTotalForceZ=off  SenseTotalTorque=off  SenseTotalTorqueX=off  SenseTotalTorqueY=off  SenseTotalTorqueZ=off  CompositeWrenchDir=FollowerOnBase  CompositeWrenchFrame=BaseFrame  EquilibriumPosition=0  EquilibriumPositionUnits=deg  SpringStiffness=0  SpringStiffnessUnits=N*m/deg  DampingCoefficient=0  DampingCoefficientUnits=kg*m^2/(rad*s)  TorqueActuationMode=InputTorque  MotionActuationMode=ComputedMotion  SensePosition=on  SenseVelocity=on  SenseAcceleration=on  SenseTorqueForce=off  SenseLowerLimitTorqueForce=off  SenseUpperLimitTorqueForce=off  LowerLimitSpecify=on  LowerLimitBound=-0.97  LowerLimitBoundUnits=rad  LowerLimitStiffness=1e4  LowerLimitStiffnessUnits=N*m/deg  LowerLimitDamping=10  LowerLimitDampingUnits=N*m/(deg/s)  LowerLimitTransitionRegionWidth=0.1  LowerLimitTransitionRegionWidthUnits=deg  UpperLimitSpecify=on  UpperLimitBound=3.14  UpperLimitBoundUnits=rad  UpperLimitStiffness=1e4  UpperLimitStiffnessUnits=N*m/deg  UpperLimitDamping=10  UpperLimitDampingUnits=N*m/(deg/s)  UpperLimitTransitionRegionWidth=0.1  UpperLimitTransitionRegionWidthUnits=deg  PositionTargetSpecify=on  PositionTargetPriority=High  PositionTargetValue=q0(4)  PositionTargetValueUnits=rad  VelocityTargetSpecify=on  VelocityTargetPriority=High  VelocityTargetValue=dq0(4)  VelocityTargetValueUnits=deg/s
  Rev3 : sm_lib/Joints/Revolute Joint  JointMode=Normal  SenseConstraintForce=off  SenseConstraintForceX=off  SenseConstraintForceY=off  SenseConstraintForceZ=off  SenseConstraintTorque=off  SenseConstraintTorqueX=off  SenseConstraintTorqueY=off  SenseConstraintTorqueZ=off  SenseTotalForce=off  SenseTotalForceX=off  SenseTotalForceY=off  SenseTotalForceZ=off  SenseTotalTorque=off  SenseTotalTorqueX=off  SenseTotalTorqueY=off  SenseTotalTorqueZ=off  CompositeWrenchDir=FollowerOnBase  CompositeWrenchFrame=BaseFrame  EquilibriumPosition=0  EquilibriumPositionUnits=deg  SpringStiffness=0  SpringStiffnessUnits=N*m/deg  DampingCoefficient=0  DampingCoefficientUnits=kg*m^2/(rad*s)  TorqueActuationMode=InputTorque  MotionActuationMode=ComputedMotion  SensePosition=on  SenseVelocity=on  SenseAcceleration=on  SenseTorqueForce=off  SenseLowerLimitTorqueForce=off  SenseUpperLimitTorqueForce=off  LowerLimitSpecify=on  LowerLimitBound=-1.55  LowerLimitBoundUnits=rad  LowerLimitStiffness=1e4  LowerLimitStiffnessUnits=N*m/deg  LowerLimitDamping=10  LowerLimitDampingUnits=N*m/(deg/s)  LowerLimitTransitionRegionWidth=0.1  LowerLimitTransitionRegionWidthUnits=deg  UpperLimitSpecify=on  UpperLimitBound=1.57  UpperLimitBoundUnits=rad  UpperLimitStiffness=1e4  UpperLimitStiffnessUnits=N*m/deg  UpperLimitDamping=10  UpperLimitDampingUnits=N*m/(deg/s)  UpperLimitTransitionRegionWidth=0.1  UpperLimitTransitionRegionWidthUnits=deg  PositionTargetSpecify=on  PositionTargetPriority=High  PositionTargetValue=q0(3)  PositionTargetValueUnits=rad  VelocityTargetSpecify=on  VelocityTargetPriority=High  VelocityTargetValue=dq0(3)  VelocityTargetValueUnits=rad/s
  Rev7 : sm_lib/Joints/Revolute Joint  JointMode=Normal  SenseConstraintForce=off  SenseConstraintForceX=off  SenseConstraintForceY=off  SenseConstraintForceZ=off  SenseConstraintTorque=off  SenseConstraintTorqueX=off  SenseConstraintTorqueY=off  SenseConstraintTorqueZ=off  SenseTotalForce=off  SenseTotalForceX=off  SenseTotalForceY=off  SenseTotalForceZ=off  SenseTotalTorque=off  SenseTotalTorqueX=off  SenseTotalTorqueY=off  SenseTotalTorqueZ=off  CompositeWrenchDir=FollowerOnBase  CompositeWrenchFrame=BaseFrame  EquilibriumPosition=0  EquilibriumPositionUnits=deg  SpringStiffness=0  SpringStiffnessUnits=N*m/deg  DampingCoefficient=0  DampingCoefficientUnits=kg*m^2/(rad*s)  TorqueActuationMode=InputTorque  MotionActuationMode=ComputedMotion  SensePosition=on  SenseVelocity=on  SenseAcceleration=on  SenseTorqueForce=off  SenseLowerLimitTorqueForce=off  SenseUpperLimitTorqueForce=off  LowerLimitSpecify=on  LowerLimitBound=-1.57  LowerLimitBoundUnits=rad  LowerLimitStiffness=1e4  LowerLimitStiffnessUnits=N*m/deg  LowerLimitDamping=10  LowerLimitDampingUnits=N*m/(deg/s)  LowerLimitTransitionRegionWidth=0.1  LowerLimitTransitionRegionWidthUnits=deg  UpperLimitSpecify=on  UpperLimitBound=1.57  UpperLimitBoundUnits=rad  UpperLimitStiffness=1e4  UpperLimitStiffnessUnits=N*m/deg  UpperLimitDamping=10  UpperLimitDampingUnits=N*m/(deg/s)  UpperLimitTransitionRegionWidth=0.1  UpperLimitTransitionRegionWidthUnits=deg  PositionTargetSpecify=on  PositionTargetPriority=High  PositionTargetValue=q0(1)  PositionTargetValueUnits=rad  VelocityTargetSpecify=on  VelocityTargetPriority=High  VelocityTargetValue=dq0(1)  VelocityTargetValueUnits=rad/s
  Rigid9 : sm_lib/Joints/Weld Joint  JointMode=Normal  SenseConstraintForce=off  SenseConstraintForceX=off  SenseConstraintForceY=off  SenseConstraintForceZ=off  SenseConstraintTorque=off  SenseConstraintTorqueX=off  SenseConstraintTorqueY=off  SenseConstraintTorqueZ=off  SenseTotalForce=off  SenseTotalForceX=off  SenseTotalForceY=off  SenseTotalForceZ=off  SenseTotalTorque=off  SenseTotalTorqueX=off  SenseTotalTorqueY=off  SenseTotalTorqueZ=off  CompositeWrenchDir=FollowerOnBase  CompositeWrenchFrame=BaseFrame
  SPS tau_Actuator{1..7} (7 alike) : nesl_utility/Simulink-PS Converter  Commented=on  PhysicalDomain=network_engine_domain  SubClassName=ps_input  LeftPortType=input  RightPortType=output  PseudoPeriodic=off  Frequencies=[]  NoiseDistribution=none  NoiseParameters=[]  Unit=1  AffineConversion=off  FilteringAndDerivatives=provide  SimscapeFilterOrder=1  InputFilterTimeConstant=0.001  UdotUserProvided=0
      settings: SourceProductBaseCode=SS,PW,VE
  SPS tau_Actuator{8..11} (4 alike) : nesl_utility/Simulink-PS Converter  PhysicalDomain=network_engine_domain  SubClassName=ps_input  LeftPortType=input  RightPortType=output  PseudoPeriodic=off  Frequencies=[]  NoiseDistribution=none  NoiseParameters=[]  Unit=1  AffineConversion=off  FilteringAndDerivatives=provide  SimscapeFilterOrder=1  InputFilterTimeConstant=0.001  UdotUserProvided=0
      settings: SourceProductBaseCode=SS,PW,VE
  Shoulder_Link : Subsystem  Commented=on
  Solver Configuration : nesl_utility/Solver Configuration  Commented=on  PhysicalDomain=network_engine_domain  SubClassName=solver  LeftPortType=input  RightPortType=generic  Tones=[]  Harmonics=[]  SimulateNoise=off  Profile=off  UseLocalSampling=off  EnableSwitchedLinearOptims=on  FrequencyDomain=off  UseCCode=off  RelTol=0.001  AbsTol=0.001  MinStep=1e-09  ToWorkspace=off  RevertToSquareIcSolve=off  NumHomotopyIterations=100  PhasorMode=off  PhasorModeNumHarmonics=1  IndexReductionMethod=DerivativeReplacement  DoDC=off  ResidualTolerance=1e-09  UseLocalSolver=off  LocalSolverChoice=NE_BACKWARD_EULER_ADVANCER  LocalSolverSampleTime=0.001  DoFixedCost=off  MaxNonlinIter=3  MaxModeIter=2  ComputeImpulses=off  ImpulseIterations=2  LinearAlgebra=auto  LinearAlgebraNumThread=0  EquationFormulation=NE_TIME_EF  DelaysMemoryBudget=1024  AutomaticFiltering=on  FilteringTimeConstant=0.001  PartitionStorageMethod=AS_NEEDED  PartitionMemoryBudget=1024  PartitionMethod=ROBUST
      settings: SourceProductBaseCode=SS,PW,VE
  Solver Configuration1 : nesl_utility/Solver Configuration  PhysicalDomain=network_engine_domain  SubClassName=solver  LeftPortType=input  RightPortType=generic  Tones=[]  Harmonics=[]  SimulateNoise=off  Profile=off  UseLocalSampling=off  EnableSwitchedLinearOptims=on  FrequencyDomain=off  UseCCode=off  RelTol=0.001  AbsTol=0.001  MinStep=1e-09  ToWorkspace=off  RevertToSquareIcSolve=off  NumHomotopyIterations=100  PhasorMode=off  PhasorModeNumHarmonics=1  IndexReductionMethod=DerivativeReplacement  DoDC=off  ResidualTolerance=1e-09  UseLocalSolver=off  LocalSolverChoice=NE_BACKWARD_EULER_ADVANCER  LocalSolverSampleTime=0.001  DoFixedCost=off  MaxNonlinIter=3  MaxModeIter=2  ComputeImpulses=off  ImpulseIterations=2  LinearAlgebra=auto  LinearAlgebraNumThread=0  EquationFormulation=NE_TIME_EF  DelaysMemoryBudget=1024  AutomaticFiltering=on  FilteringTimeConstant=0.001  PartitionStorageMethod=AS_NEEDED  PartitionMemoryBudget=1024  PartitionMethod=ROBUST
      settings: SourceProductBaseCode=SS,PW,VE
  World : sm_lib/Frames and Transforms/World Frame  Commented=on
  World1 : sm_lib/Frames and Transforms/World Frame
  Wrist1_Link : Subsystem  Commented=on
  Wrist2_Link : Subsystem  Commented=on
  base_link : Subsystem  Commented=on
  base_link1 : Subsystem
  tau_Demux : Demux
  Q_out : Outport
  Qdot_out : Outport  Port=2
  Qddot_out : Outport  Port=3
  wires:
  PSS Qdot_Actuator6/1 -> Goto_Qdot_Actuator6/1
  tau_Demux/2 -> [tau_Actuator2]
  From_tau_Actuator7/1 -> SPS tau_Actuator7/1
  [Qdot_Actuator4] -> Qdot_State Mux/4
  From_tau_Actuator6/1 -> SPS tau_Actuator6/1
  PSS Q_Actuator5/1 -> Goto_Q_Actuator5/1
  From_tau_Actuator1/1 -> SPS tau_Actuator1/1
  PSS Q_Actuator6/1 -> Goto_Q_Actuator6/1
  [Qddot_Actuator1] -> Qddot_State Mux/1
  From_tau_Actuator2/1 -> SPS tau_Actuator2/1
  [Qddot_Actuator3] -> Qddot_State Mux/3
  [Qdot_Actuator3] -> Qdot_State Mux/3
  [Qddot_Actuator2] -> Qddot_State Mux/2
  tau_Demux/4 -> [tau_Actuator4]
  PSS Qddot_Actuator5/1 -> Goto_Qddot_Actuator5/1
  PSS Q_Actuator3/1 -> Goto_Q_Actuator3/1
  PSS Qdot_Actuator3/1 -> Goto_Qdot_Actuator3/1
  [Q_Actuator3] -> Q_State Mux/3
  PSS Qddot_Actuator7/1 -> Goto_Qddot_Actuator7/1
  tau_Demux/1 -> [tau_Actuator1]
  tau_Demux/3 -> [tau_Actuator3]
  Qddot_State Mux/1 -> Qddot_out/1
  PSS Qdot_Actuator7/1 -> Goto_Qdot_Actuator7/1
  PSS Qddot_Actuator2/1 -> Goto_Qddot_Actuator2/1
  PSS Qddot_Actuator6/1 -> Goto_Qddot_Actuator6/1
  PSS Q_Actuator7/1 -> Goto_Q_Actuator7/1
  [Qdot_Actuator2] -> Qdot_State Mux/2
  PSS Qdot_Actuator5/1 -> Goto_Qdot_Actuator5/1
  [Q_Actuator4] -> Q_State Mux/4
  [Qddot_Actuator4] -> Qddot_State Mux/4
  [Q_Actuator2] -> Q_State Mux/2
  From_tau_Actuator4/1 -> SPS tau_Actuator4/1
  [Q_Actuator1] -> Q_State Mux/1
  From_tau_Actuator5/1 -> SPS tau_Actuator5/1
  Qdot_State Mux/1 -> Qdot_out/1
  From_tau_Actuator3/1 -> SPS tau_Actuator3/1
  Q_State Mux/1 -> Q_out/1
  [Qdot_Actuator1] -> Qdot_State Mux/1
  PSS Q_Actuator4/1 -> Goto_Q_Actuator4/1
  tau_in/1 -> tau_Demux/1
  PSS Q_Actuator1/1 -> Goto_Q_Actuator1/1
  PSS Qdot_Actuator1/1 -> Goto_Qdot_Actuator1/1
  PSS Qddot_Actuator1/1 -> Goto_Qddot_Actuator1/1
  PSS Q_Actuator2/1 -> Goto_Q_Actuator2/1
  PSS Qdot_Actuator2/1 -> Goto_Qdot_Actuator2/1
  PSS Qdot_Actuator4/1 -> Goto_Qdot_Actuator4/1
  PSS Qddot_Actuator4/1 -> Goto_Qddot_Actuator4/1
  PSS Qddot_Actuator3/1 -> Goto_Qddot_Actuator3/1
  PSS Qddot_Actuator8/1 -> [Qddot_Actuator1]
  PSS Qdot_Actuator8/1 -> [Qdot_Actuator1]
  PSS Q_Actuator8/1 -> [Q_Actuator1]
  PSS Q_Actuator9/1 -> [Q_Actuator2]
  PSS Qddot_Actuator9/1 -> [Qddot_Actuator2]
  PSS Qdot_Actuator9/1 -> [Qdot_Actuator2]
  PSS Qddot_Actuator10/1 -> [Qddot_Actuator3]
  PSS Qdot_Actuator10/1 -> [Qdot_Actuator3]
  PSS Q_Actuator10/1 -> [Q_Actuator3]
  PSS Qdot_Actuator11/1 -> [Qdot_Actuator4]
  PSS Qddot_Actuator11/1 -> [Qddot_Actuator4]
  PSS Q_Actuator11/1 -> [Q_Actuator4]
  [tau_Actuator1] -> SPS tau_Actuator8/1
  [tau_Actuator2] -> SPS tau_Actuator9/1
  [tau_Actuator3] -> SPS tau_Actuator10/1
  [tau_Actuator4] -> SPS tau_Actuator11/1
  connections:
  Actuator5/RConn2 -- PSS Q_Actuator5/LConn1
  SPS tau_Actuator4/RConn1 -- Actuator4/LConn2
  Actuator6/RConn2 -- PSS Q_Actuator6/LConn1
  SPS tau_Actuator1/RConn1 -- Actuator1/LConn2
  Actuator7/RConn3 -- PSS Qdot_Actuator7/LConn1
  Actuator6/RConn3 -- PSS Qdot_Actuator6/LConn1
  SPS tau_Actuator7/RConn1 -- Actuator7/LConn2
  Actuator3/RConn4 -- PSS Qddot_Actuator3/LConn1
  Actuator5/RConn4 -- PSS Qddot_Actuator5/LConn1
  Actuator5/RConn3 -- PSS Qdot_Actuator5/LConn1
  EndEffector_Link/LConn1 -- Endeffector/RConn1
  SPS tau_Actuator2/RConn1 -- Actuator2/LConn2
  MechanismConfiguration/RConn1 -- World/RConn1 -- base_link/LConn1 -- Solver Configuration/RConn1
  SPS tau_Actuator3/RConn1 -- Actuator3/LConn2
  Actuator4/RConn4 -- PSS Qddot_Actuator4/LConn1
  Actuator3/RConn1 -- HalfArm2_Link/LConn1
  Actuator7/RConn4 -- PSS Qddot_Actuator7/LConn1
  Actuator6/RConn4 -- PSS Qddot_Actuator6/LConn1
  Actuator7/RConn2 -- PSS Q_Actuator7/LConn1
  Actuator2/RConn1 -- HalfArm1_Link/LConn1
  SPS tau_Actuator5/RConn1 -- Actuator5/LConn2
  SPS tau_Actuator6/RConn1 -- Actuator6/LConn2
  Actuator3/RConn3 -- PSS Qdot_Actuator3/LConn1
  Actuator2/RConn4 -- PSS Qddot_Actuator2/LConn1
  Actuator4/RConn2 -- PSS Q_Actuator4/LConn1
  Actuator1/LConn1 -- base_link/RConn1
  Actuator7/RConn1 -- Bracelet_Link/LConn1
  Actuator2/LConn1 -- Shoulder_Link/RConn1
  Actuator7/LConn1 -- Wrist2_Link/RConn1
  Bracelet_Link/RConn1 -- Endeffector/LConn1
  Actuator5/RConn1 -- Wrist1_Link/LConn1
  Actuator5/LConn1 -- ForeArm_Link/RConn1
  Actuator3/LConn1 -- HalfArm1_Link/RConn1
  Actuator4/RConn1 -- ForeArm_Link/LConn1
  Actuator4/LConn1 -- HalfArm2_Link/RConn1
  Actuator6/RConn1 -- Wrist2_Link/LConn1
  Actuator1/RConn1 -- Shoulder_Link/LConn1
  Actuator6/LConn1 -- Wrist1_Link/RConn1
  Actuator1/RConn2 -- PSS Q_Actuator1/LConn1
  Actuator1/RConn3 -- PSS Qdot_Actuator1/LConn1
  Actuator1/RConn4 -- PSS Qddot_Actuator1/LConn1
  Actuator2/RConn2 -- PSS Q_Actuator2/LConn1
  Actuator2/RConn3 -- PSS Qdot_Actuator2/LConn1
  Actuator3/RConn2 -- PSS Q_Actuator3/LConn1
  Actuator4/RConn3 -- PSS Qdot_Actuator4/LConn1
  Solver Configuration1/RConn1 -- MechanismConfiguration1/RConn1 -- World1/RConn1 -- base_link1/LConn1
  Mid_Arm_Solidbody_v2_1/LConn1 -- Rev3/RConn1
  Gripper_Arm_Solidbody_v2_1/LConn1 -- Rev11/RConn1
  Rev7/LConn1 -- base_link1/RConn1
  Lower_Arm_Solidbody_v2_1/RConn1 -- Rev3/LConn1
  Base_Gear_Solidbody_v3_1/LConn1 -- Rev7/RConn1
  Gripper_Dumb_Solid_v1_1/LConn1 -- Rigid9/RConn1
  Lower_Arm_Solidbody_v2_1/LConn1 -- Rev10/RConn1
  Base_Gear_Solidbody_v3_1/RConn1 -- Rev10/LConn1
  Mid_Arm_Solidbody_v2_1/RConn1 -- Rev11/LConn1
  Gripper_Arm_Solidbody_v2_1/RConn1 -- Rigid9/LConn1
  PSS Qddot_Actuator8/LConn1 -- Rev7/RConn4
  PSS Qdot_Actuator8/LConn1 -- Rev7/RConn2
  PSS Q_Actuator8/LConn1 -- Rev7/RConn3
  PSS Qddot_Actuator9/LConn1 -- Rev10/RConn4
  PSS Qdot_Actuator9/LConn1 -- Rev10/RConn3
  PSS Q_Actuator9/LConn1 -- Rev10/RConn2
  PSS Qddot_Actuator10/LConn1 -- Rev3/RConn4
  PSS Qdot_Actuator10/LConn1 -- Rev3/RConn3
  PSS Q_Actuator10/LConn1 -- Rev3/RConn2
  PSS Q_Actuator11/LConn1 -- Rev11/RConn2
  PSS Qddot_Actuator11/LConn1 -- Rev11/RConn4
  PSS Qdot_Actuator11/LConn1 -- Rev11/RConn3
  SPS tau_Actuator8/RConn1 -- Rev7/LConn2
  SPS tau_Actuator9/RConn1 -- Rev10/LConn2
  SPS tau_Actuator10/RConn1 -- Rev3/LConn2
  SPS tau_Actuator11/RConn1 -- Rev11/LConn2

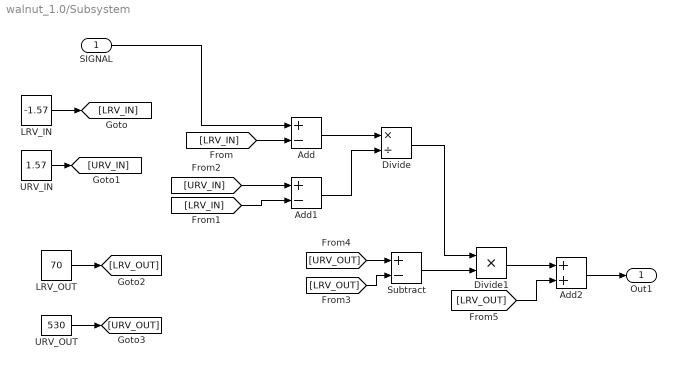
== system walnut_1.0/Subsystem ==
  SIGNAL : Inport
  Add : Sum  Inputs=+-
  Add1 : Sum  Inputs=+-
  Add2 : Sum
  Divide : Product  Inputs=*/
  Divide1 : Product
  LRV_IN : Constant  Value=-1.57
  LRV_OUT : Constant  Value=70
  Subtract : Sum  Inputs=+-
  URV_IN : Constant  Value=1.57
  URV_OUT : Constant  Value=530
  Out1 : Outport
  wires:
  SIGNAL/1 -> Add/1
  LRV_IN/1 -> [LRV_IN]
  URV_IN/1 -> [URV_IN]
  [LRV_IN] -> Add/2
  [LRV_IN] -> Add1/2
  [URV_IN] -> Add1/1
  Add/1 -> Divide/1
  Add1/1 -> Divide/2
  LRV_OUT/1 -> [LRV_OUT]
  URV_OUT/1 -> [URV_OUT]
  Divide/1 -> Divide1/1
  Subtract/1 -> Divide1/2
  Add2/1 -> Out1/1
  Divide1/1 -> Add2/1
  [LRV_OUT] -> Subtract/2
  [URV_OUT] -> Subtract/1
  [LRV_OUT] -> Add2/2

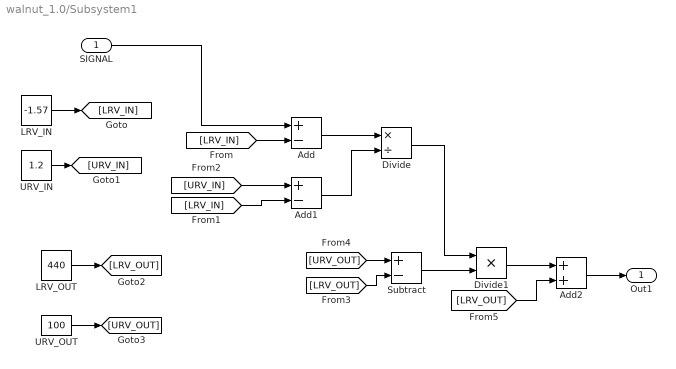
== system walnut_1.0/Subsystem1 ==
  SIGNAL : Inport
  Add : Sum  Inputs=+-
  Add1 : Sum  Inputs=+-
  Add2 : Sum
  Divide : Product  Inputs=*/
  Divide1 : Product
  LRV_IN : Constant  Value=-1.57
  LRV_OUT : Constant  Value=440
  Subtract : Sum  Inputs=+-
  URV_IN : Constant  Value=1.2
  URV_OUT : Constant  Value=100
  Out1 : Outport
  wires:
  SIGNAL/1 -> Add/1
  LRV_IN/1 -> [LRV_IN]
  URV_IN/1 -> [URV_IN]
  [LRV_IN] -> Add/2
  [LRV_IN] -> Add1/2
  [URV_IN] -> Add1/1
  Add/1 -> Divide/1
  Add1/1 -> Divide/2
  LRV_OUT/1 -> [LRV_OUT]
  URV_OUT/1 -> [URV_OUT]
  Divide/1 -> Divide1/1
  Subtract/1 -> Divide1/2
  Add2/1 -> Out1/1
  Divide1/1 -> Add2/1
  [LRV_OUT] -> Subtract/2
  [URV_OUT] -> Subtract/1
  [LRV_OUT] -> Add2/2

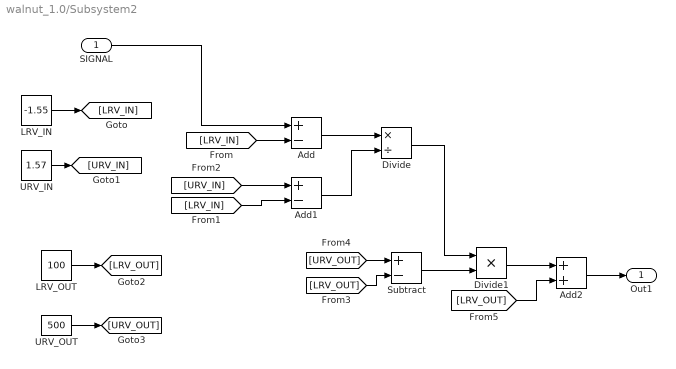
== system walnut_1.0/Subsystem2 ==
  SIGNAL : Inport
  Add : Sum  Inputs=+-
  Add1 : Sum  Inputs=+-
  Add2 : Sum
  Divide : Product  Inputs=*/
  Divide1 : Product
  LRV_IN : Constant  Value=-1.55
  LRV_OUT : Constant  Value=100
  Subtract : Sum  Inputs=+-
  URV_IN : Constant  Value=1.57
  URV_OUT : Constant  Value=500
  Out1 : Outport
  wires:
  SIGNAL/1 -> Add/1
  LRV_IN/1 -> [LRV_IN]
  URV_IN/1 -> [URV_IN]
  [LRV_IN] -> Add/2
  [LRV_IN] -> Add1/2
  [URV_IN] -> Add1/1
  Add/1 -> Divide/1
  Add1/1 -> Divide/2
  LRV_OUT/1 -> [LRV_OUT]
  URV_OUT/1 -> [URV_OUT]
  Divide/1 -> Divide1/1
  Subtract/1 -> Divide1/2
  Add2/1 -> Out1/1
  Divide1/1 -> Add2/1
  [LRV_OUT] -> Subtract/2
  [URV_OUT] -> Subtract/1
  [LRV_OUT] -> Add2/2

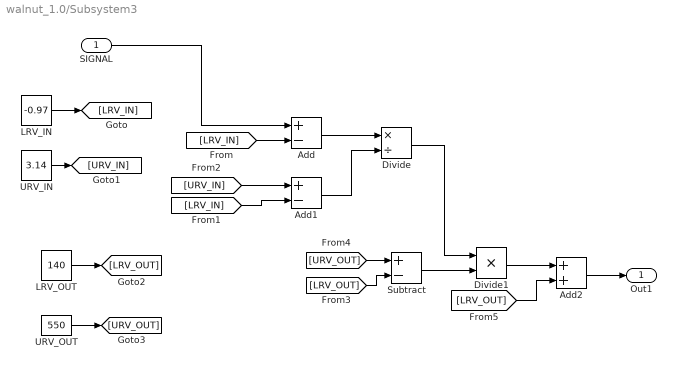
== system walnut_1.0/Subsystem3 ==
  SIGNAL : Inport
  Add : Sum  Inputs=+-
  Add1 : Sum  Inputs=+-
  Add2 : Sum
  Divide : Product  Inputs=*/
  Divide1 : Product
  LRV_IN : Constant  Value=-0.97
  LRV_OUT : Constant  Value=140
  Subtract : Sum  Inputs=+-
  URV_IN : Constant  Value=3.14
  URV_OUT : Constant  Value=550
  Out1 : Outport
  wires:
  SIGNAL/1 -> Add/1
  LRV_IN/1 -> [LRV_IN]
  URV_IN/1 -> [URV_IN]
  [LRV_IN] -> Add/2
  [LRV_IN] -> Add1/2
  [URV_IN] -> Add1/1
  Add/1 -> Divide/1
  Add1/1 -> Divide/2
  LRV_OUT/1 -> [LRV_OUT]
  URV_OUT/1 -> [URV_OUT]
  Divide/1 -> Divide1/1
  Subtract/1 -> Divide1/2
  Add2/1 -> Out1/1
  Divide1/1 -> Add2/1
  [LRV_OUT] -> Subtract/2
  [URV_OUT] -> Subtract/1
  [LRV_OUT] -> Add2/2
